simulink model "c6711dskANC_hsrtdx"  (Simulink 6.0)
settings: Solver=FixedStepDiscrete  StartTime=0.0  StopTime=inf  RelTol=1e-3
libraries: c6711dsklib x3, rtdxBlocks x3, dspsrcs4 x3, dspbuff3 x1, c6000tgtpreflib x1, adapt_frame x1, dsparch4 x1
settings Model: Creator=navan  LastModifiedBy=thartley  ProdHWDeviceType=TI C6000
settings DataIOCC: LimitDataPoints=off  SaveOutput=off  SaveTime=off  SignalLoggingName=sigsOut
settings OptimizationCC: InlineParams=on  InlineInvariantSignals=off
settings DebuggingCC: CheckExecutionContextPreStartOutputMsg=on  CheckExecutionContextRuntimeOutputMsg=on  SolverPrmCheckMsg=none
settings HardwareCC: ProdBitPerLong=40  ProdEndianess=LittleEndian  ProdHWDeviceType=TI C6000  TargetHWDeviceType=32-bit Generic
settings ModelReferenceCC: UpdateModelReferenceTargets=IfOutOfDate
settings RTWCC: SystemTargetFile=ti_c6000.tlc  GenCodeOnly=on  TemplateMakefile=ti_c6000.tmf  ProcessScript=ti_c6000_make_rtw_hook
settings STFCustomTargetCC: TargetFcnLib=ansi_tfl_tmw.mat  MatFileLogging=on  LifeSpan=inf  SystemTargetFile=ti_c6000.tlc  ActivateCallback=c6000_callback('ActivateCallback',hSrc,hDlg);
settings GRTTargetCC: ModelReferenceCompliant=off  LifeSpan=inf
settings CustomProperty: DataType=RTWOptions_EnumType_S__A_matlab_toolbox_rtw_targets_tic6000_tic6000_ti_c6000_BoardType  Value=C6711DSK
settings EnumStrPairs: String=C6416DSK
settings SFSimCC: SFSimApplyToAllLibs=on  SFSimBuildMode=Incremental

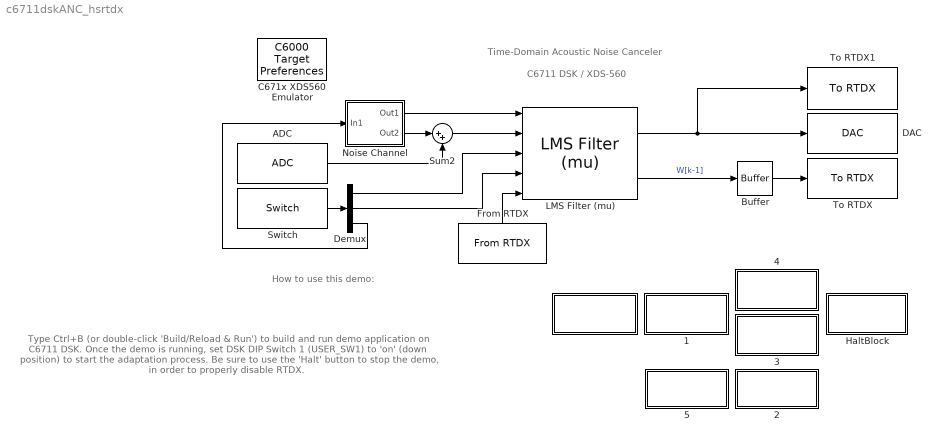
== system c6711dskANC_hsrtdx ==
  note: Time-Domain Acoustic Noise Canceler
  note: C6711 DSK / XDS-560
  note: Type Ctrl+B (or double-click 'Build/Reload & Run')
      | to build and run demo application on C6711 DSK.
      |
      | Once the demo is running, set DSK DIP Switch 1
      | (USER_SW1) to 'on' (down position) to start the
      | adaptation process.
      |
      | Be sure to use the 'Halt' button to stop the demo, in order
      | to properly disable RTDX.
  note: How to use this demo:
  " " : Subsystem
      settings: OpenFcn=ANC_script('run')
      mask Type: Run demo
      mask Display: disp(sprintf('Build / Reload\n& Run'))
  " 1" : Subsystem
      settings: OpenFcn=ANC_script('RTDX')
      mask Type: Run demo
      mask Display: disp(sprintf('Display\n RTDX Data'))
  " 2" : Subsystem
      settings: OpenFcn=edit ANC_script
      mask Type: Run demo
      mask Description: Double-clicking this button will display the demo script which generates code, builds, loads, executes application on the DSP, and arbitrates RTDX transfers.
      mask Display: disp(sprintf('View Demo \nScript'))
  " 3" : Subsystem
      settings: OpenFcn=ANC_script('change_mu',0.001);
      mask Display: disp('Slow\nAdapt')
  " 4" : Subsystem
      settings: OpenFcn=ANC_script('change_mu',0.04);
      mask Display: disp('Fast\nAdapt')
  " 5" : Subsystem
      settings: OpenFcn=web(fullfile(matlabroot,'toolbox','rtw','targets','tic6000','tic6000demos','html','ANC_doc.html'))
      mask Type: Run demo
      mask Description: Double-clicking this button will display the demo script which generates code, builds, loads, executes application on the DSP, and arbitrates RTDX transfers.
      mask Display: disp('Info')
  ADC : c6711dsklib/ADC  ADCsource=Line In  MicGain=off  OutputDataType=Single  Scaling=Normalize  SourceGain=0.0  FrameSize=256
  Buffer : dspbuff3/Buffer  N=8  V=0  ic=0
  C671x XDS560 Emulator : c6000tgtpreflib/C6000 Target Preferences
  DAC : c6711dsklib/DAC  Scaling=Normalize  DacAtten=0.0  OverflowMode=Wrap
  Demux : Demux  Outputs=3
  From RTDX : rtdxBlocks/From RTDX  Orientation=up  channelNameStr=iMu  isBlocking=off  icMaskVar=0.001  Ts=256/8000  dims=[1 1]  isFrame=off  dType=single  isChannelEnabled=off  isHighSpeedRTDXUsed=on
  HaltBlock : Subsystem  AncestorBlock=c6711dsklib/Reset
      settings: OpenFcn=ANC_script('halt')
      mask Display: disp('Halt Demo');
  LMS Filter (mu) : adapt_frame/LMS Filter (mu)  N=32  leakage=1.0
  Noise Channel : Subsystem
  Sum2 : Sum  Inputs=|++  SaturateOnIntegerOverflow=on  InputSameDT=on
  Switch : c6711dsklib/Switch  sw1=off  sw2=on  sw3=off  dType=Boolean  Ts=256/8000
  To RTDX : rtdxBlocks/To RTDX  channelNameStr=outTaps  isChannelEnabled=off
  To RTDX1 : rtdxBlocks/To RTDX  channelNameStr=Err  isChannelEnabled=off
  wires:
  LMS Filter (mu)/1 -> DAC/1, To RTDX1/1
  ADC/1 -> Sum2/2
  Noise Channel/2(Out2) -> Sum2/1
  Sum2/1 -> LMS Filter (mu)/2
  Switch/1 -> Demux/1
  Demux/1 -> LMS Filter (mu)/3
  Demux/2 -> LMS Filter (mu)/4
  Buffer/1 -> To RTDX/1
  Noise Channel/1(Out1) -> LMS Filter (mu)/1
  Demux/3 -> Noise Channel/1(In1)
  From RTDX/1 -> LMS Filter (mu)/5
  LMS Filter (mu)/2 -> Buffer/1  "W[k-1]"

== system c6711dskANC_hsrtdx/  ==

== system c6711dskANC_hsrtdx/ 1 ==

== system c6711dskANC_hsrtdx/ 2 ==

== system c6711dskANC_hsrtdx/ 3 ==

== system c6711dskANC_hsrtdx/ 4 ==

== system c6711dskANC_hsrtdx/ 5 ==

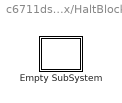
== system c6711dskANC_hsrtdx/HaltBlock ==
  Empty SubSystem : Subsystem

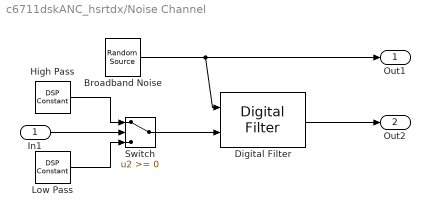
== system c6711dskANC_hsrtdx/Noise Channel ==
  In1 : Inport
  Broadband Noise : dspsrcs4/Random Source  SrcType=Gaussian  NormMethod=Sum of uniform values  CltLength=5  Min=0  Max=1  Mean=0  Var=0.2  RepMode=Specify seed  Seed=[23341]  Inherit=off  SampMode=Discrete  SampTime=1/8000  SampFrame=256  DataType=Single  OutComplex=Real
  Digital Filter : dsparch4/Digital Filter  TypePopup=FIR (all zeros)  IIRFiltStruct=Direct form II transposed  AllPoleFiltStruct=Direct form  FIRFiltStruct=Direct form  CoeffSource=Input port(s)  NumCoeffs=[1 2]  DenCoeffs=[1 0.1]  BiQuadCoeffs=[1 0.3 0.4 1 0.1 0.2]  LatticeCoeffs=[0.2 0.4]  denIgnore=on  FiltPerSampPopup=One filter per frame  IC=0  ICnum=0  ICden=0  roundingMode=Floor  overflowMode=off
  High Pass : dspsrcs4/DSP Constant  Value=single([0.00493427189488606 -0.00596085391438248 -0.0100028665950744 0.000247624247658316 0.0136346086248442 0.00499735400511394 -0.0189539275340475 -0.0168748387438599 0.0203757595600775 0.035365951918637 -0.0143987965290339 -0.0640193820794684 -0.00860427731620416 0.118290255249928 0.0991576384227279 -0.491423287322378 0.491423287322378 -0.0991576384227279 -0.118290255249928 0.00860427731620416 0.0640193820794684 0.0143987965290339 -0.035365951918637 -0.0203757595600775 0.0168748387438599 0.0189539275340475 -0.00499735400511394 -0.0136346086248442 -0.000247624247658316 0.0100028665950744 0.00596085391438248 -0.00493427189488606])  SampleMode=Discrete  discreteOutput=Sample-based  continuousOutput=Sample-based  sampTime=256/8000  framePeriod=2  dataType=Inherit from 'Constant value'  wordLen=16  udDataType=sfix(16)  fracBitsMode=Best precision  numFracBits=15  InterpretAs1D=-inf  Ts=-inf  FramebasedOutput=-inf
  Low Pass : dspsrcs4/DSP Constant  Value=single([0.00134550092740892 0.000523816682121889 0.00420303599278532 0.00632655262041013 -0.0143222876697505 -0.0389824015898802 -0.0103937897059368 0.0478667359432575 0.0407952413345009 -0.00403845698847935 0.0264625284266877 0.0517683541033748 -0.0922904697037772 -0.235175831919441 -0.0585231709321379 0.273497649258539 0.273497649258539 -0.0585231709321379 -0.235175831919441 -0.0922904697037772 0.0517683541033748 0.0264625284266877 -0.00403845698847935 0.0407952413345009 0.0478667359432575 -0.0103937897059368 -0.0389824015898802 -0.0143222876697505 0.00632655262041013 0.00420303599278532 0.000523816682121889 0.00134550092740892])  SampleMode=Discrete  discreteOutput=Sample-based  continuousOutput=Sample-based  sampTime=256/8000  framePeriod=2  dataType=Inherit from 'Constant value'  wordLen=16  udDataType=sfix(16)  fracBitsMode=Best precision  numFracBits=15  InterpretAs1D=-inf  Ts=-inf  FramebasedOutput=-inf
  Switch : Switch  SaturateOnIntegerOverflow=on
  Out1 : Outport
  Out2 : Outport  Port=2
  wires:
  Broadband Noise/1 -> Out1/1, Digital Filter/1
  Digital Filter/1 -> Out2/1
  Switch/1 -> Digital Filter/2
  High Pass/1 -> Switch/1
  Low Pass/1 -> Switch/3
  In1/1 -> Switch/2

== system c6711dskANC_hsrtdx/HaltBlock/Empty SubSystem ==
